simulink model "Ejer12_AlcoholSangre"  (R2023b)
settings: Solver=VariableStepAuto  StartTime=0.0  StopTime=10.0  RelTol=1e-3
undefined symbols (not defined in the file): d
settings Model: Creator=alfre  LastModifiedBy=alfre

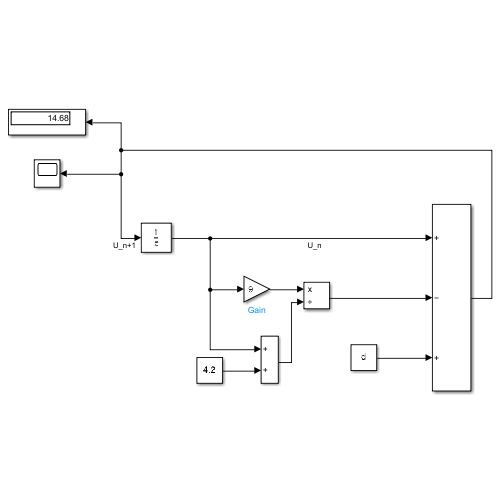
[thumbnail: Simulink's stored preview of the top-level diagram]
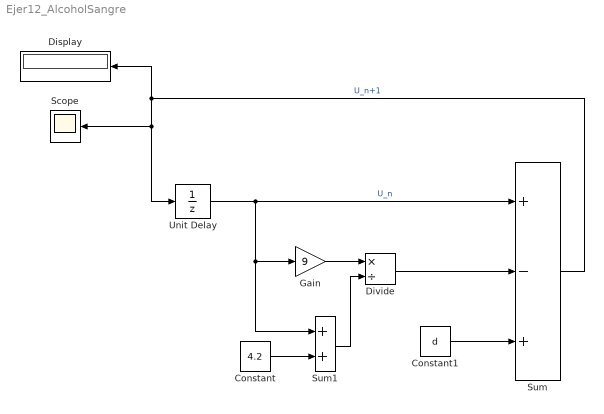
== system Ejer12_AlcoholSangre ==
  Constant : Constant  Value=4.2
  Constant1 : Constant  Value=d
  Display : Display
  Divide : Product  Inputs=*/
  Gain : Gain  Gain=9
  Scope : Scope
  Sum : Sum  Inputs=+-+
  Sum1 : Sum
  Unit Delay : UnitDelay  SampleTime=-1  HasFrameUpgradeWarning=on
  wires:
  Unit Delay/1 -> Sum/1, Sum1/1, Gain/1  "U_n"
  Sum/1 -> Display/1, Unit Delay/1, Scope/1  "U_n+1"
  Gain/1 -> Divide/1
  Constant/1 -> Sum1/2
  Sum1/1 -> Divide/2
  Divide/1 -> Sum/2
  Constant1/1 -> Sum/3
